simulink subsystem "StreetLaneSegment2x1_BUS_asSubsystem"  (R2021a)
settings: Solver=VariableStepAuto  StartTime=0.0  StopTime=10.0  RelTol=1e-3
undefined symbols (not defined in the file): x0z, xz, yin, yout, yz
libraries: StreetLanesLibrary x1
settings Model: Creator=phill  LastModifiedBy=phill

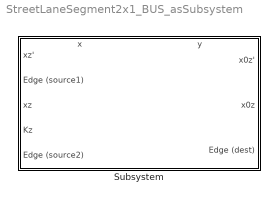
== system StreetLaneSegment2x1_BUS_asSubsystem ==
  Subsystem : Subsystem  mask{Kz=0, Tz=0}
      mask prompts: Kz "Kz (Capacity - How many cars fit into this cell)"; Tz "Tz (Nominal travel time for vehicles traveling unobstructed through the cell)"
      mask help: The 2x1 version of the basic 1x1 cell
      settings: PortSchema="{\"entries\":[{\"content\":{\"sides\":[{\"content\":{\"connectorIds\":[\"Out5\",\"In1\",\"Out6\",\"Out7\",\"In2\"]},\"type\":\"ConnectorPlacement.EquallySpacedRectSide\",\"uuid\":\"95d0121f-acb2-4e25-97c7-15db8ac80d70\"},{\"content\":{\"connectorIds\":[\"Out1\",\"Out2\",\"In3\"],\"side\":\"RIGHT\"},\"type\":\"ConnectorPlacement.EquallySpacedRectSide\",\"uuid\":\"74008a0d-3aff-4b45-b66c-7df902aff109\"},{\"content\":{\"connectorIds\":[\"Out3\",\"Out4\"],\"side\":\"TOP\"},\"type\":\"ConnectorPlacement.EquallySpacedRectSide\",\"uuid\":\"60b01591-4a61-43c7-92fb-9786f4f21d2e\"}]},\"type\":\"ConnectorPlacement.EquallySpacedConnector\",\"uuid\":\"7f6ca8c0-19be-43e0-a232-af4f67956fb4\"}],\"packageUris\":[\"http://schema.mathworks.com/mf0/Connector/R2020b\"],\"version\":\"1.0\"}"
      mask Display:
      | image('$imagefile'); % Use "Edit Image" on toolstrip to change.
      | disp('Street Lane Segment 2x1 \n\n');
      | disp(['Kz = ', get_param(gcb,'Kz'), ' | Tz = ', get_param(gcb, 'Tz')])

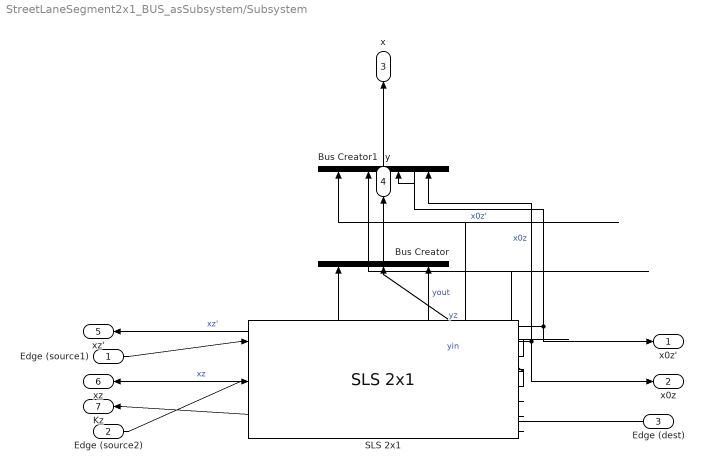
== system StreetLaneSegment2x1_BUS_asSubsystem/Subsystem ==
  Edge (source1) : Inport
  Edge (source2) : Inport  Port=2
  Edge (dest) : Inport  Port=3
  Bus Creator : BusCreator  Inputs=yin,yz,yout
  Bus Creator1 : BusCreator  Inputs=xz,xz',x0z',x0z
  SLS 2x1 : StreetLanesLibrary/SLS 2x1  Kz=0  Tz=0
  x0z' : Outport
  x0z : Outport  Port=2
  x : Outport  Port=3
  y : Outport  Port=4
  xz' : Outport  Port=5
  xz : Outport  Port=6
  Kz : Outport  Port=7
  wires:
  SLS 2x1/3 -> Bus Creator/1  "yin"
  SLS 2x1/2 -> x0z/1, Bus Creator1/4  "x0z"
  SLS 2x1/7 -> xz/1, Bus Creator1/1  "xz"
  SLS 2x1/1 -> x0z'/1, Bus Creator1/3  "x0z'"
  Bus Creator/1 -> y/1
  Edge (source1)/1 -> SLS 2x1/1
  Bus Creator1/1 -> x/1
  SLS 2x1/5 -> Bus Creator/3  "yout"
  SLS 2x1/6 -> xz'/1, Bus Creator1/2  "xz'"
  SLS 2x1/8 -> Kz/1
  SLS 2x1/4 -> Bus Creator/2  "yz"
  Edge (source2)/1 -> SLS 2x1/2
  Edge (dest)/1 -> SLS 2x1/3
